simulink model "simple"  (Simulink 8.7)
settings: Solver=VariableStepDiscrete  StartTime=0.0  StopTime=10.0  RelTol=1e-3
settings Model: Creator=arnaud  LastModifiedBy=Teme
settings DataIOCC: SaveFormat=Structure  SignalLoggingSaveFormat=ModelDataLogs
settings OptimizationCC: ExpressionDepthLimit=2147483647
settings DebuggingCC: SolverPrmCheckMsg=warning  FcnCallInpInsideContextMsg=UseLocalSettings  StateNameClashWarn=warning  StrictBusMsg=Warning
settings GRTTargetCC: CombineOutputUpdateFcns=off  GRTInterface=on
settings ConfigComp: CovSFcnEnable=off

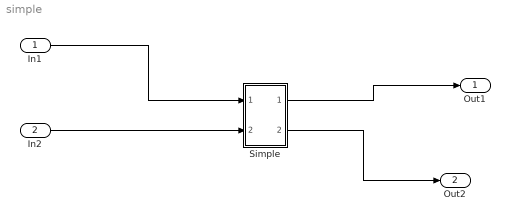
== system simple ==
  In1 : Inport
  In2 : Inport  Port=2
  "Simple " : Subsystem
  Out1 : Outport
  Out2 : Outport  Port=2
  wires:
  In1/1 -> "Simple "/1(In1)
  In2/1 -> "Simple "/2(In2)
  "Simple "/1(Out1) -> Out1/1
  "Simple "/2(Out2) -> Out2/1

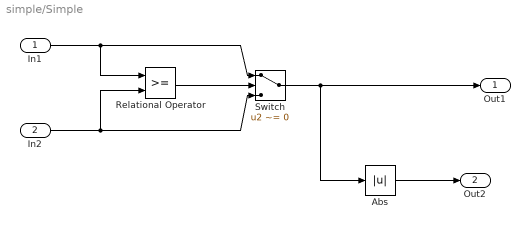
== system simple/Simple  ==
  In1 : Inport
  In2 : Inport  Port=2
  Abs : Abs
  Relational Operator : RelationalOperator  OutDataTypeStr=boolean
  Switch : Switch  Criteria=u2 ~= 0
  Out1 : Outport
  Out2 : Outport  Port=2
  wires:
  Switch/1 -> Out1/1, Abs/1
  Abs/1 -> Out2/1
  In1/1 -> Relational Operator/1, Switch/1
  Relational Operator/1 -> Switch/2
  In2/1 -> Relational Operator/2, Switch/3
